simulink model "Steering_Column_test"  (R2023a)
settings: Solver=VariableStepAuto  StartTime=0.0  StopTime=10.0  RelTol=1e-3
InitFcn:
  | [modelDir, ~, ~] = fileparts(get_param(bdroot, 'FileName'));
  | run(fullfile(modelDir, 'startup_project.m'));
settings Model: Creator=Tan_Tram  LastModifiedBy=Tan_Tram

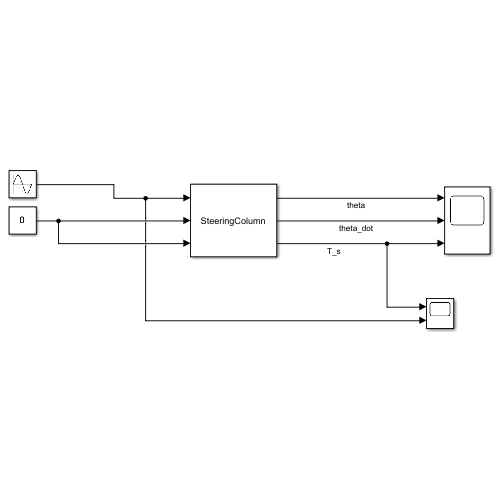
[thumbnail: Simulink's stored preview of the top-level diagram]
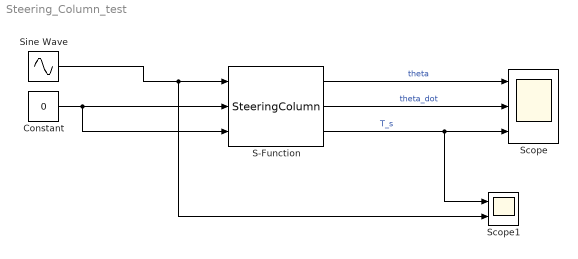
== system Steering_Column_test ==
  Constant : Constant  Value=0
  S-Function : S-Function  FunctionName=SteeringColumn  Parameters=p.J_total, p.B_total, p.T_f_total  SFunctionDeploymentMode=off  EnableBusSupport=off
  Scope : Scope  NumInputPorts=3
  Scope1 : Scope  NumInputPorts=2
  Sine Wave : Sin  Amplitude=3  SampleTime=0
  wires:
  Sine Wave/1 -> Scope1/2, S-Function/1
  Constant/1 -> S-Function/3, S-Function/2
  S-Function/1 -> Scope/1  "theta"
  S-Function/3 -> Scope1/1, Scope/3  "T_s"
  S-Function/2 -> Scope/2  "theta_dot"
